simulink model "Helicopter"  (R2021b)
settings: Solver=VariableStepAuto  StartTime=0.0  StopTime=137  RelTol=1e-3
values from neighbouring files (symbols this model uses):
  A = double(subs(A_lin, [x;u], [x_s;u_s]))    [Linearize.m]
  a_B = lsqcurvefit(fun,x0,U,F_B)    [Motor_Chara.m]
  a_F = lsqcurvefit(fun,x0,U,F_F)    [Motor_Chara.m]
  B = double(subs(B_lin, [x;u], [x_s;u_s]))    [Linearize.m]
  C = [eye(3), zeros(3,3)]    [Linearize.m]
  D = zeros(3,2)    [Linearize.m]
  Flimit = ulimit.^2*(a_F+a_B)/2    [Controller.m]
  K = K(:,1:8)    [Controller.m]
  L = place(A',C', -1*[1.05, 1.1, 1.2, 1.3, 1.4, 1.5]*max_eig_ctrl)'    [Controller.m]
  l_1 = 495e-3    (= 0.495)    [Param.m]
  l_2 = 177.5e-3    (= 0.1775)    [Param.m]
  l_3 = 210e-3    (= 0.21)    [Param.m]
  l_4 = 228.5e-3    (= 0.2285)    [Param.m]
  l_5 = 135.5e-3    (= 0.1355)    [Param.m]
  l_6 = 262e-3    (= 0.262)    [Param.m]
  l_7 = 655e-3    (= 0.655)    [Param.m]
  l_8 = 51.5e-3    (= 0.0515)    [Param.m]
  l_H = 915e-3    (= 0.915)    [Param.m]
  m_B = 0.487    [Param.m]
  m_F = 0.487    [Param.m]
  m_H = 0.377    [Param.m]
  m_J = 0.202    [Param.m]
  m_N = 0.138    [Param.m]
  m_S = 0.322    [Param.m]
  m_W = 1.918    [Param.m]
  phi = deg2rad(15)    [Param.m]
  u_s = double([F_F_stat;F_B_stat])    [Linearize.m]
  x_0 = [0;deg2rad(-27);0;0;0;0]    [Linearize.m]
  x_s = [0;-phi;0;0;0;0]    [Linearize.m]
  y_s = C*x_s    [Linearize.m]
undefined symbols (not defined in the file or in its folder): HIL, System
libraries: quarc_library x4
settings Model: Creator=w_yuj  LastModifiedBy=w_yuj

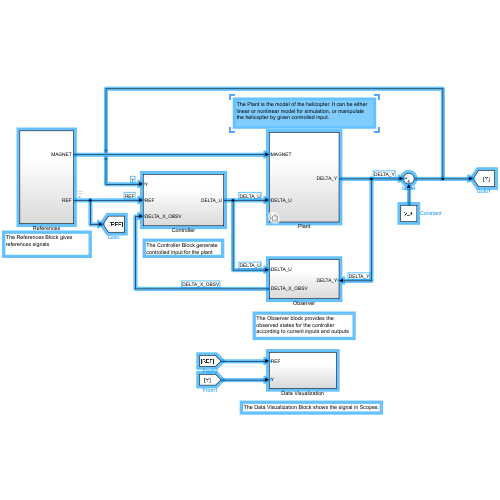
[thumbnail: Simulink's stored preview of the top-level diagram]
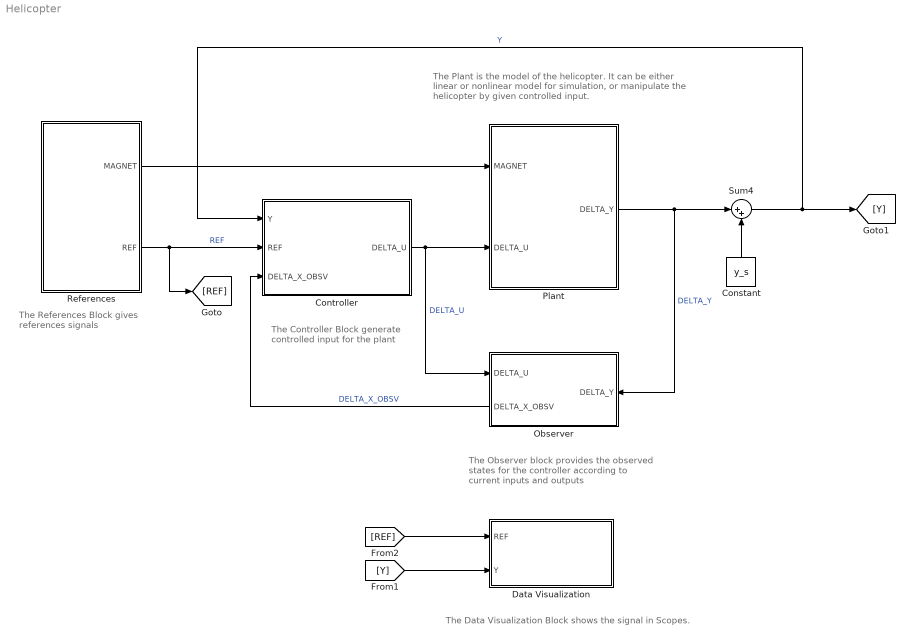
== system Helicopter ==
  note: The Observer block provides the observed states for the controller according to current inputs and outputs
  note: The Controller Block generate controlled input for the plant
  note: The Data Visualization Block shows the signal in Scopes.
  note: The References Block gives references signals
  note: The Plant is the model of the helicopter. It can be either linear or nonlinear model for simulation, or manipulate the helicopter by given controlled input.
  Constant : Constant  Value=y_s
  Controller : Subsystem
  Data Visualization : Subsystem
  Observer : Subsystem
      settings: PortSchema="{\"entries\":[{\"content\":{\"sides\":[{\"content\":{\"connectorIds\":[\"In1\"]},\"type\":\"ConnectorPlacement.EquallySpacedRectSide\",\"uuid\":\"84bc8a13-99f6-408d-b313-faa7d6e991a2\"},{\"content\":{\"connectorIds\":[\"In2\",\"Out1\"],\"side\":\"RIGHT\"},\"type\":\"ConnectorPlacement.EquallySpacedRectSide\",\"uuid\":\"d8597314-a5ac-4644-8793-325f8fc169ed\"},{\"content\":{\"connectorIds\":[],\"side\":\"TOP\"},\"type\":\"ConnectorPlacement.EquallySpacedRectSide\",\"uuid\":\"b622f082-6370-4210-b09a-1ae417550683\"}]},\"type\":\"ConnectorPlacement.EquallySpacedConnector\",\"uuid\":\"1b5549db-7ec0-46c3-874c-ec463577dbaf\"}],\"packageUris\":[\"http://schema.mathworks.com/mf0/Connector/R2020b\"],\"version\":\"1.0\"}"
  Plant : Subsystem  Variant=on
  References : Subsystem
  Sum4 : Sum  Inputs=|++
  wires:
  References/2(REF) -> [REF], Controller/2(REF)  "REF"
  Sum4/1 -> Controller/1(Y), [Y]  "Y"
  [REF] -> Data Visualization/1(REF)
  [Y] -> Data Visualization/2(Y)
  Controller/1(DELTA_U) -> Plant/2(DELTA_U), Observer/2(DELTA_U)  "DELTA_U"
  Observer/1(DELTA_X_OBSV) -> Controller/3(DELTA_X_OBSV)  "DELTA_X_OBSV"
  Plant/1(DELTA_Y) -> Observer/1(DELTA_Y), Sum4/1  "DELTA_Y"
  Constant/1 -> Sum4/2
  References/1(MAGNET) -> Plant/1(MAGNET)

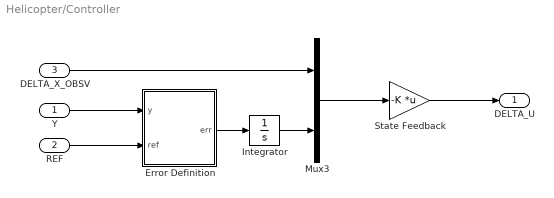
== system Helicopter/Controller ==
  Y : Inport
  REF : Inport  Port=2
  DELTA_X_OBSV : Inport  Port=3
  Error Definition : MATLAB Function  TreatAsAtomicUnit=on
  Integrator : Integrator
  Mux3 : Mux  Inputs=2
  State Feedback : Gain  Gain=-K  Multiplication=Matrix(K*u)
  DELTA_U : Outport
  wires:
  Integrator/1 -> Mux3/2
  State Feedback/1 -> DELTA_U/1
  Mux3/1 -> State Feedback/1
  Error Definition/1(err) -> Integrator/1
  Y/1 -> Error Definition/1(y)
  REF/1 -> Error Definition/2(ref)
  DELTA_X_OBSV/1 -> Mux3/1

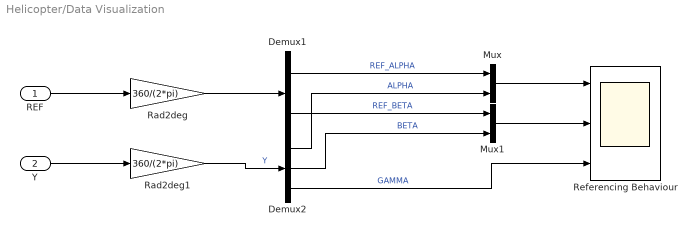
== system Helicopter/Data Visualization ==
  REF : Inport
  Y : Inport  Port=2
  Demux1 : Demux  Outputs=2
  Demux2 : Demux  Outputs=3
  Mux : Mux  Inputs=2
  Mux1 : Mux  Inputs=2
  Rad2deg : Gain  Gain=360/(2*pi)
      mask Display: disp("rad2deg")
  Rad2deg1 : Gain  Gain=360/(2*pi)
      mask Display: disp("rad2deg")
  Referencing Behaviour : Scope  NumInputPorts=3
  wires:
  Rad2deg/1 -> Demux1/1
  Y/1 -> Rad2deg1/1
  REF/1 -> Rad2deg/1
  Rad2deg1/1 -> Demux2/1  "Y"
  Mux/1 -> Referencing Behaviour/1
  Mux1/1 -> Referencing Behaviour/2
  Demux1/1 -> Mux/1  "REF_ALPHA"
  Demux2/1 -> Mux/2  "ALPHA"
  Demux1/2 -> Mux1/1  "REF_BETA"
  Demux2/2 -> Mux1/2  "BETA"
  Demux2/3 -> Referencing Behaviour/3  "GAMMA"

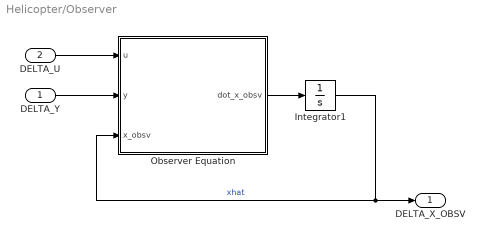
== system Helicopter/Observer ==
  DELTA_Y : Inport
  DELTA_U : Inport  Port=2
  Integrator1 : Integrator  InitialCondition=x_0-x_s
  Observer Equation : MATLAB Function  TreatAsAtomicUnit=on
  DELTA_X_OBSV : Outport
  wires:
  Integrator1/1 -> Observer Equation/3(x_obsv), DELTA_X_OBSV/1  "xhat"
  DELTA_U/1 -> Observer Equation/1(u)
  DELTA_Y/1 -> Observer Equation/2(y)
  Observer Equation/1(dot_x_obsv) -> Integrator1/1

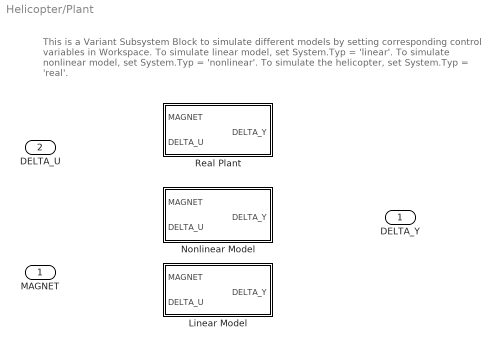
== system Helicopter/Plant ==
  note: This is a Variant Subsystem Block to simulate different models by setting corresponding control variables in Workspace. To simulate linear model, set System.Typ = 'linear'. To simulate nonlinear model, set System.Typ = 'nonlinear'. To simulate the helicopter, set System.Typ = 'real'.
  MAGNET : Inport
  DELTA_U : Inport  Port=2
  Linear Model : Subsystem  VariantControl=strcmp(System.Typ,'linear')
  Nonlinear Model : Subsystem  VariantControl=strcmp(System.Typ,'nonlinear')
  Real Plant : Subsystem  VariantControl=strcmp(System.Typ,'real')
  DELTA_Y : Outport

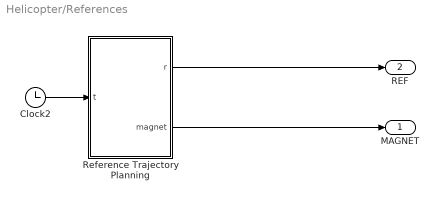
== system Helicopter/References ==
  Clock2 : Clock
  Reference Trajectory Planning : MATLAB Function  TreatAsAtomicUnit=on
  MAGNET : Outport
  REF : Outport  Port=2
  wires:
  Clock2/1 -> Reference Trajectory Planning/1(t)
  Reference Trajectory Planning/2(magnet) -> MAGNET/1
  Reference Trajectory Planning/1(r) -> REF/1

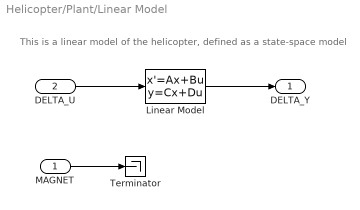
== system Helicopter/Plant/Linear Model ==
  note: This is a linear model of the helicopter, defined as a state-space model
  MAGNET : Inport
  DELTA_U : Inport  Port=2
  Linear Model : StateSpace  A=A  B=B  C=C  D=D  InitialCondition=0
  Terminator : Terminator
  DELTA_Y : Outport
  wires:
  Linear Model/1 -> DELTA_Y/1
  DELTA_U/1 -> Linear Model/1
  MAGNET/1 -> Terminator/1

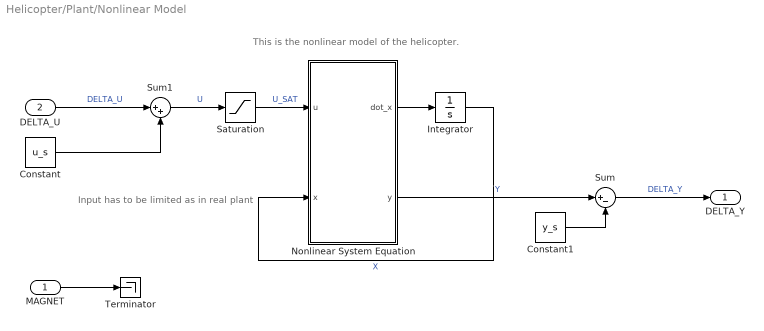
== system Helicopter/Plant/Nonlinear Model ==
  note: Input has to be limited as in real plant
  note: This is the nonlinear model of the helicopter.
  MAGNET : Inport
  DELTA_U : Inport  Port=2
  Constant : Constant  Value=u_s
  Constant1 : Constant  Value=y_s
  Integrator : Integrator  InitialCondition=x_0
  Nonlinear System Equation : MATLAB Function  TreatAsAtomicUnit=on
  Saturation : Saturate  UpperLimit=Flimit  LowerLimit=0
  Sum : Sum  Inputs=|+-
  Sum1 : Sum  Inputs=|++
  Terminator : Terminator
  DELTA_Y : Outport
  wires:
  DELTA_U/1 -> Sum1/1  "DELTA_U"
  Sum1/1 -> Saturation/1  "U"
  Constant/1 -> Sum1/2
  Nonlinear System Equation/2(y) -> Sum/1  "Y"
  Sum/1 -> DELTA_Y/1  "DELTA_Y"
  Nonlinear System Equation/1(dot_x) -> Integrator/1
  Constant1/1 -> Sum/2
  Saturation/1 -> Nonlinear System Equation/1(u)  "U_SAT"
  Integrator/1 -> Nonlinear System Equation/2(x)  "X"
  MAGNET/1 -> Terminator/1

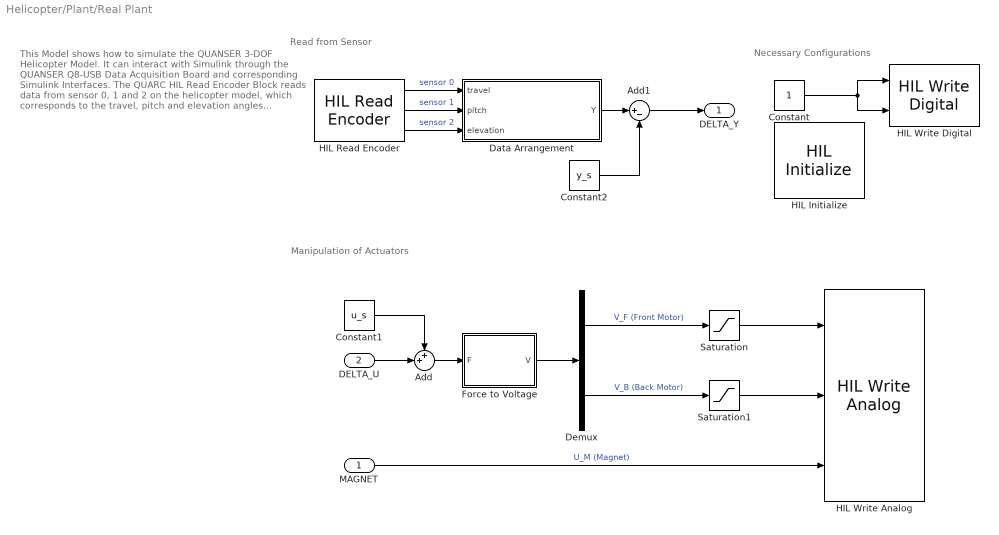
== system Helicopter/Plant/Real Plant ==
  note: This Model shows how to simulate the QUANSER 3-DOF Helicopter Model. It can interact with Simulink through the QUANSER Q8-USB Data Acquisition Board and corresponding Simulink Interfaces.
      |
      | The QUARC HIL Read Encoder Block reads data from sensor 0, 1 and 2 on the helicopter model, which corresponds to the travel, pitch and elevation angles respectively. Through Data Arrangement Block will these measured numbers be translated into real angle in rad, and be combined as the output vector Y.
      |
      | The QUARC HIL Write Analog Block set voltages of the front and back motors, as well as the voltage of the electric magnet, according to its input signals.
      |
      | The QUARC HIL Initialize Block is necessary for the initialization of the system. The QUARC HIL Write Digital is to activate or deactivate the Amplifier, where in this model we activate it as default.
  note: Manipulation of Actuators
  note: Read from Sensor
  note: Necessary Configurations
  MAGNET : Inport
  DELTA_U : Inport  Port=2
  Add : Sum  Inputs=++|
  Add1 : Sum  Inputs=|+-
  Constant : Constant
  Constant1 : Constant  Value=u_s
  Constant2 : Constant  Value=y_s
  "Data Arrangement " : Subsystem
  Demux : Demux  Outputs=2
  Force to Voltage : MATLAB Function  TreatAsAtomicUnit=on
  HIL Initialize : quarc_library/Data Acquisition/Generic/Configuration/HIL Initialize  object_name=HIL-1  board_type=q8_usb  board_number=0  board_options=update_rate=normal;decimation=1  exclusive=off  active=on  hardware_clocks=[0:2]  clock_modes=[]  initial_clock_frequencies=[]  set_clock_params_at_start=off  set_clock_params_at_switch_in=off  set_clock_frequencies_at_start=off  set_clock_frequencies_at_switch_in=off  analog_input_channels=[0:7]  analog_input_configurations=[]  analog_input_maximums=10  analog_input_minimums=-10  set_analog_input_params_at_start=on  set_analog_input_params_at_switch_in=off  analog_output_channels=[0:7]  analog_output_maximums=10  analog_output_minimums=-10  initial_analog_outputs=[0]  final_analog_outputs=[0]  watchdog_analog_outputs=0  set_analog_output_params_at_start=on  set_analog_output_params_at_switch_in=off  set_analog_outputs_at_start=on  set_analog_outputs_at_switch_in=off  set_analog_outputs_at_terminate=on  set_analog_outputs_at_switch_out=off  set_analog_outputs_on_watchdog=off  digital_input_channels=[]  digital_output_channels=[]  digital_output_configuration=[]  initial_digital_outputs=[1]  final_digital_outputs=[1]  watchdog_digital_outputs=[1]  set_digital_output_params_at_start=off  set_digital_output_params_at_switch_in=off  set_digital_outputs_at_start=on  set_digital_outputs_at_switch_in=off  set_digital_outputs_at_terminate=on  set_digital_outputs_at_switch_out=off  set_digital_outputs_on_watchdog=off  encoder_channels=[0:7]  quadrature=[4]  encoder_filter_frequency=[]  initial_encoder_counts=[0]  set_encoder_params_at_start=on  set_encoder_params_at_switch_in=off  set_encoder_counts_at_start=on  set_encoder_counts_at_switch_in=off  pwm_channels=[0:7]  pwm_modes=0  pwm_frequency=99.532799999999995e6/4095  pwm_configuration=[0]  pwm_alignment=[0]  pwm_polarity=[1]  pwm_leading_deadband=[0]  pwm_trailing_deadband=[0]  initial_pwm_outputs=[0]  final_pwm_outputs=[0]  watchdog_pwm_outputs=[0]  set_pwm_params_at_start=on  set_pwm_params_at_switch_in=off  set_pwm_outputs_at_start=on  set_pwm_outputs_at_switch_in=off  set_pwm_outputs_at_terminate=on  set_pwm_outputs_at_switch_out=off  set_pwm_outputs_on_watchdog=off  other_output_channels=[]  initial_other_outputs=[]  final_other_outputs=[]  watchdog_other_outputs=[]  set_other_outputs_at_start=off  set_other_outputs_at_switch_in=off  set_other_outputs_at_terminate=off  set_other_outputs_at_switch_out=off  set_other_outputs_on_watchdog=off
  HIL Read Encoder : quarc_library/Data Acquisition/Generic/Immediate I//O/HIL Read Encoder  object_name=HIL-1  channels=[0;1;2]  sample_time=qc_get_step_size  active=on  vector_output=off  data_type_mode=Inherit via back propagation  data_type=double
  HIL Write Analog : quarc_library/Data Acquisition/Generic/Immediate I//O/HIL Write Analog  object_name=HIL-1  channels=[0;1;2]  sample_time=-1  active=off  vector_input=off
  HIL Write Digital : quarc_library/Data Acquisition/Generic/Immediate I//O/HIL Write Digital  object_name=HIL-1  channels=[0;1]  sample_time=-1  active=off  vector_input=off
      settings: SourceProductName=QUARC Targets
  Saturation : Saturate  UpperLimit=4  LowerLimit=0
  Saturation1 : Saturate  UpperLimit=4  LowerLimit=0
  DELTA_Y : Outport
  wires:
  Add/1 -> Force to Voltage/1(F)
  "Data Arrangement "/1(Y) -> Add1/1
  DELTA_U/1 -> Add/2
  Force to Voltage/1(V) -> Demux/1
  Constant2/1 -> Add1/2
  Constant1/1 -> Add/1
  Saturation1/1 -> HIL Write Analog/2
  Demux/2 -> Saturation1/1  "V_B (Back Motor)"
  HIL Read Encoder/2 -> "Data Arrangement "/2(pitch)  "sensor 1"
  Add1/1 -> DELTA_Y/1
  HIL Read Encoder/1 -> "Data Arrangement "/1(travel)  "sensor 0"
  Demux/1 -> Saturation/1  "V_F (Front Motor)"
  MAGNET/1 -> HIL Write Analog/3  "U_M (Magnet)"
  Constant/1 -> HIL Write Digital/1, HIL Write Digital/2
  HIL Read Encoder/3 -> "Data Arrangement "/3(elevation)  "sensor 2"
  Saturation/1 -> HIL Write Analog/1

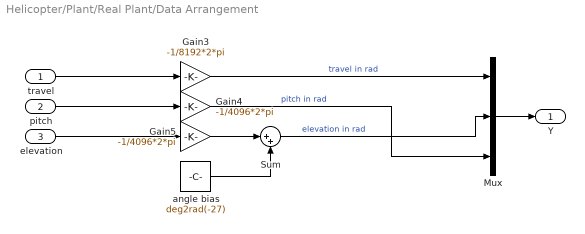
== system Helicopter/Plant/Real Plant/Data Arrangement  ==
  travel : Inport
  pitch : Inport  Port=2
  elevation : Inport  Port=3
  Gain3 : Gain  Gain=-1/8192*2*pi
  Gain4 : Gain  Gain=-1/4096*2*pi
  Gain5 : Gain  Gain=-1/4096*2*pi
  Mux : Mux  Inputs=3
  Sum : Sum  Inputs=|++
  angle bias : Constant  Value=deg2rad(-27)
  Y : Outport
  wires:
  Gain3/1 -> Mux/1  "travel in rad"
  angle bias/1 -> Sum/2
  Gain5/1 -> Sum/1
  travel/1 -> Gain3/1
  pitch/1 -> Gain4/1
  elevation/1 -> Gain5/1
  Mux/1 -> Y/1
  Sum/1 -> Mux/2  "elevation in rad"
  Gain4/1 -> Mux/3  "pitch in rad"

== matlab function Helicopter/Observer/Observer Equation ==
  data: u input; y input; x_obsv input; dot_x_obsv output; A parameter; B parameter; C parameter; L parameter
function dot_x_obsv = obsv(u, y, x_obsv, A, B, C, L)

dot_x_obsv = A*x_obsv + B*u + L*(y - C*x_obsv);

== matlab function Helicopter/References/Reference Trajectory Planning ==
  data: t input; r output; magnet output
function [r,magnet] = traj(t)

    timearray =[10, 15, 25, 30, 35 ,40, 60, 70, 76, 86, 110, 115, 125, 130];
    % Punkte
    r_0 = [0;deg2rad(-27)];                     % Punkt 0
    r_1 = [0;deg2rad(0)];
    r_2 = [90*pi/180; deg2rad(0)];
    r_21 =[90*pi/180; deg2rad(-10.5)];
    r_3 = [90*pi/180; deg2rad(-20)];
    r_4 = [90*pi/180; deg2rad(0)];
    r_5 = [450*pi/180; deg2rad(0)];
    r_6 = [450*pi/180; deg2rad(-18)];
    r_7 = [450*pi/180; deg2rad(0)];
    r_8 = [0*pi/180; deg2rad(0)];
    r_9 = [0*pi/180; deg2rad(-20)];
    r_10 = [0*pi/180; deg2rad(-25)];

    % Trajektorie
    if t<=timearray(1) 
        r = (r_1-r_0)./timearray(1)*(t-0)+r_0;
        %r = r_1;                            % Punkt 0-1
        magnet = 0;
    elseif t < timearray(2)
        r = (r_2-r_1)./(timearray(2)-timearray(1))*(t-timearray(1))+r_1;       % Punkt 1-2
        magnet = 0;
    elseif t < timearray(3)
        r = r_2;                            % Punkt 2 
        magnet = 0;
        
    elseif t < timearray(4)
        r = r_21;
        magnet = 0;
    elseif t < timearray(5) 
        r = r_3;                            % Punkt 3 (Magnet aufnehmen)
        magnet = 1;
    elseif t < timearray(6) 
        r = r_4;                            % Punkt 4
        magnet = 1;
    elseif t < timearray(7)
        r = (r_5-r_4)./(timearray(7)-timearray(6))*(t-timearray(6))+r_4;      % Punkt 4-5
        magnet = 1;
    elseif t < timearray(8)
        r = r_5;                            % Punkt 5
        magnet = 1;
    elseif t < timearray(9)
        r = r_6;                            % Punkt 6
        magnet = 1;
    elseif t < timearray(10) 
        r = r_7;                            % Punkt 7
        magnet = 0;
    elseif t < timearray(11)
        r = (r_8-r_7)./(timearray(11)-timearray(10))*(t-timearray(10))+r_7;      % Punkt 7-8
        magnet = 0;
    elseif t < timearray(12) 
        r = r_8;                            % Punkt 8
        magnet = 0;
    elseif t < timearray(13) 
        r = r_9;                            % Punkt 9
        magnet = 0;
    elseif t < timearray(14)
        r = r_10;     % Punkt 9-10
        magnet = 0;
    else
        r = r_10;
        magnet = 0;
    end
end

== matlab function Helicopter/Plant/Nonlinear Model/Nonlinear System Equation ==
  data: u input size=2,1; dot_x output size=6,1; x input size=6,1; y output; m_S parameter; m_F parameter; m_B parameter; m_H parameter; m_N parameter; m_W parameter; m_J parameter; l_1 parameter; l_2 parameter; l_3 parameter; l_4 parameter; l_5 parameter; l_6 parameter; l_7 parameter; l_8 parameter; l_H parameter; phi parameter
%Dies ist die die Funktion zur Berechnung der Ableitung des Zustandsvektors
%dx 
%
%Eingänge:
%Motorkräfte F_F, F_F
%Ausgang:
%Ableitung des Zustandsvektors dx

function [dot_x, y] = nonlin(u, x, ...
                m_S, m_F, m_B, m_H, m_N, m_W, m_J, ...
                l_1, l_2, l_3, l_4, l_5, l_6, l_7, l_8, l_H, phi)

% Gravitationsbeschleunigung
g = 9.81;

% Eingaenge - Propellerkraft:
F_F = u(1);
F_B = u(2);

% Gemessene Zustaende:
alpha = x(1);
beta  = x(2);
gamma = x(3);
dalpha = x(4);
dbeta = x(5);
dgamma = x(6);
% 
% % Eingangs Parameter
% m_S = param(1);
% m_F = param(2);
% m_B = param(3);
% m_H = param(4);
% m_N = param(5);
% m_W = param(6);
% m_J = param(7);
% 
% l_1 = param(8);
% l_2 = param(9);
% l_3 = param(10);
% l_4 = param(11);
% l_5 = param(12);
% l_6 = param(13);
% l_7 = param(14);
% l_8 = param(15);
% l_H = param(16);
% phi = param(17);

%Berechnung der Traegheitsmomente
J_x = m_H*l_H^2/12 + m_H*l_3^2 + m_N*(l_4+l_5*cos(phi))^2*cos(beta)^2 + ...
    m_W*(l_4+l_6*cos(phi))^2*cos(beta)^2 + (m_J+m_S)*l_7^2*cos(beta)^2 + ...
    (m_F+m_B)*(l_7^2*cos(beta)^2+l_2^2*cos(gamma)^2);

%%%%%%%%%%%%%%%%%%%%%%% Fehler korrigiert %%%%%%%%%%%%%%%%%%%%%%%%%%%%%%%%
% J_y = m_H*l_H^2/12 + m_H*(l_3^2 + l_8^2) + m_N*((l_4+l_5*cos(gamma))^2+...
%     (l_8-l_5*sin(gamma))^2) + m_W*((l_4+l_6*cos(gamma))^2+...
%     (l_8-l_6*sin(gamma))^2) + (m_J+m_S+m_F+m_B)*(l_7^2+l_8^2);
J_y = m_H*l_H^2/12 + l_H*(l_3^2 + l_8^2) + m_N*((l_4+l_5*cos(phi))^2+...
    (l_8-l_5*sin(phi))^2) + m_W*((l_4+l_6*cos(phi))^2+...
    (l_8-l_6*sin(phi))^2) + (m_J+m_S+m_F+m_B)*(l_7^2+l_8^2); 
%%%%%%%%%%%%%%%%%%%%%%%%%%%%%%%%%%%%%%%%%%%%%%%%%%%%%%%%%%%%%%%%%%%%%%%%%%
J_z = m_S*l_1^2/12 + (m_F+m_B)*l_2^2;

% Berechnung der Momenten
M_MOT_GAMMA = l_2*(F_F-F_B);
M_N = m_N*g*((l_4+l_5*cos(phi))*cos(beta)-l_8*sin(beta));
M_H = -m_H*g*(l_3*cos(beta)+l_8*sin(beta));
M_W = m_W*g*((l_4+l_6*cos(phi))*cos(beta)-l_8*sin(beta));
M_B = -m_B*g*(l_7*cos(beta)+l_8*sin(beta));
M_JS = -(m_J+m_S)*g*(l_7*cos(beta)+l_8*sin(beta));
M_F = -m_F*g*(l_7*cos(beta)+l_8*sin(beta));
M_MOT_BETA = l_7*(F_F+F_B)*cos(gamma);
%%% korrigiert
M_MOT_ALPHA = -l_7*(F_F+F_B)*cos(beta)*sin(gamma);


%Berechnung der Bewegungsgleichungen in Zustandsraumdarstellung
 
dot_x =  [dalpha;...        
       dbeta;...
       dgamma;...   
       M_MOT_ALPHA/J_x;...
       (M_MOT_BETA+M_N+M_H+M_W+M_B+M_JS+M_F)/J_y;...
       M_MOT_GAMMA/J_z];

y = [alpha; beta; gamma];

end

== matlab function Helicopter/Controller/Error Definition ==
  data: y input; err output; ref input
function err = error(y, ref)

err = [ref(1)-y(1); ref(2)-y(2)];

end

== matlab function Helicopter/Plant/Real Plant/Force to Voltage ==
  data: F input; V output; a_F parameter; a_B parameter
function V = force2volt(F, a_F, a_B)

V = zeros(2,1);

V(1) = 1/a_F * sqrt(F(1));
V(2) = 1/a_B * sqrt(F(2));

end
